simulink model "PassiveHydraulicPTOSim"  (R2014a)
settings: Solver=ode45  StartTime=0.0  StopTime=param.stop  FixedStep=0.0001  MaxStep=0.05  RelTol=1e-6
libraries: PTOSim_Lib x6
settings Model: Creator=sor  LastModifiedBy=sor

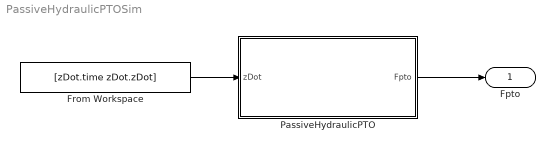
== system PassiveHydraulicPTOSim ==
  From Workspace : FromWorkspace  VariableName=[zDot.time zDot.zDot]  SampleTime=0  Interpolate=off  OutputAfterFinalValue=Holding final value
  PassiveHydraulicPTO : Subsystem
  Fpto : Outport
  wires:
  From Workspace/1 -> PassiveHydraulicPTO/1(zDot)
  PassiveHydraulicPTO/1(Fpto) -> Fpto/1

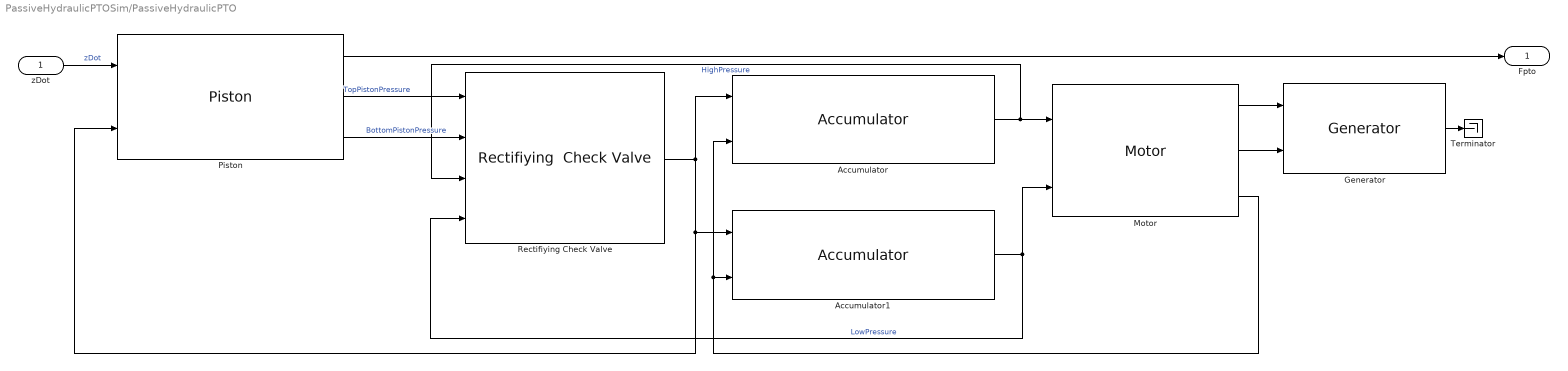
== system PassiveHydraulicPTOSim/PassiveHydraulicPTO ==
  zDot : Inport
  Accumulator : PTOSim_Lib/Hydraulic_PTO/Accumulator  OverrideUsingVariant=Variant  pto=0
  Accumulator1 : PTOSim_Lib/Hydraulic_PTO/Accumulator  OverrideUsingVariant=Variant1  pto=0
  Generator : PTOSim_Lib/Hydraulic_PTO/Generator  pto=0
  "Motor " : PTOSim_Lib/Hydraulic_PTO/Motor   pto=0
  "Piston " : PTOSim_Lib/Hydraulic_PTO/Piston    pto=0
  Rectifiying Check Valve : PTOSim_Lib/Hydraulic_PTO/Rectifiying  Check Valve  pto=0
  Terminator : Terminator
  Fpto : Outport
  wires:
  zDot/1 -> "Piston "/1  "zDot"
  "Piston "/2 -> Rectifiying Check Valve/1  "TopPistonPressure"
  "Piston "/3 -> Rectifiying Check Valve/2  "BottomPistonPressure"
  "Piston "/1 -> Fpto/1
  Accumulator/1 -> Rectifiying Check Valve/3, "Motor "/1  "HighPressure"
  Accumulator1/1 -> Rectifiying Check Valve/4, "Motor "/2  "LowPressure"
  "Motor "/3 -> Accumulator1/2, Accumulator/2
  "Motor "/1 -> Generator/1
  "Motor "/2 -> Generator/2
  Generator/1 -> Terminator/1
  Rectifiying Check Valve/1 -> Accumulator/1, "Piston "/2, Accumulator1/1
